simulink model "enumModel"  (R2016b)
settings: Solver=VariableStepAuto  StartTime=0.0  StopTime=10.0  RelTol=1e-3
undefined symbols (not defined in the file or in its folder): enum1
libraries: simulink x2
settings Model: Creator=Radwa  LastModifiedBy=Radwa

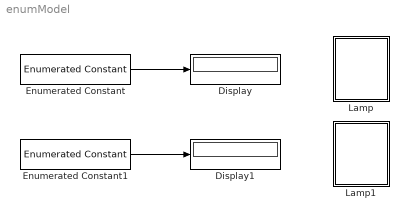
== system enumModel ==
  Display : Display
  Display1 : Display
  Enumerated Constant : simulink/Sources/Enumerated Constant  OutDataTypeStr=Enum: enum1  Value=enum1.true  SampleTime=inf
  Enumerated Constant1 : simulink/Sources/Enumerated Constant  OutDataTypeStr=Enum: enum1  Value=enum1.false  SampleTime=inf
  Lamp : Subsystem  DialogController=hmiCreateDDGDialog  IsWebBlock=on  mask(MWDashboardBlock){webBlockId=1e379ca5-ccd9-4f60-a56f-9d5289d10a7a, webBlockType=lamp, ShowInLibBrowser=on, ShowInitialText=on, HMISrcModelName=untitled}
      mask prompts: webBlockType "WebBlock Type"; HMISrcModelName "Source Model"
      mask help: SimulinkHMI:dialogs:LampDialogDesc
      mask Help: helpview([docroot '/mapfiles/simulink.map'], 'hmi_lamp')
      mask Display:
      | if strcmp(get_param(bdroot(gcb),'BlockDiagramType'), 'library')
      |     image([(matlabroot) '/toolbox/simulink/hmi/icons/Lamp.png']);
      | end
  Lamp1 : Subsystem  DialogController=hmiCreateDDGDialog  IsWebBlock=on  mask(MWDashboardBlock){webBlockId=cb7bde1c-1d15-43df-87c0-4a6af3ffcd77, webBlockType=lamp, ShowInLibBrowser=on, ShowInitialText=on, HMISrcModelName=untitled}
      mask prompts: webBlockType "WebBlock Type"; HMISrcModelName "Source Model"
      mask help: SimulinkHMI:dialogs:LampDialogDesc
      mask Help: helpview([docroot '/mapfiles/simulink.map'], 'hmi_lamp')
      mask Display:
      | if strcmp(get_param(bdroot(gcb),'BlockDiagramType'), 'library')
      |     image([(matlabroot) '/toolbox/simulink/hmi/icons/Lamp.png']);
      | end
  wires:
  Enumerated Constant/1 -> Display/1
  Enumerated Constant1/1 -> Display1/1

== system enumModel/Lamp ==

== system enumModel/Lamp1 ==
